simulink model "harvester"  (R2025b)
settings: Solver=FixedStepAuto  StartTime=0.0  StopTime=100  FixedStep=0.1  RelTol=1e-3
values from neighbouring files (symbols this model uses):
  nDrum = 1000    [Script.m]
  nEngine = 2500    [Script.m]
  nHeader = 100    [Script.m]
  sDrum = 1    [Script.m]
  sEngine = 1    [Script.m]
  sGrainConveyor = 1    [Script.m]
  sHeader = 1    [Script.m]
settings Model: Creator=levadny  LastModifiedBy=andr
settings OptimizationCC: DefaultParameterBehavior=Inlined  UseDivisionForNetSlopeComputation=on  OptimizeBlockIOStorage=off  EnhancedBackFolding=on  PassReuseOutputArgsThreshold=0.0  ZeroExternalMemoryAtStartup=off  ZeroInternalMemoryAtStartup=off  OptimizeDataStoreBuffers=off  BusAssignmentInplaceUpdate=off
settings DebuggingCC: ParameterTunabilityLossMsg=error  SFUnexpectedBacktrackingDiag=warning  SFNoUnconditionalDefaultTransitionDiag=warning
settings HardwareCC: ProdLongLongMode=on
settings SFSimCC: SimTargetLang=C++  SimDLTargetLibrary=mkl-dnn
settings RTWCC: GenerateReport=on  BuildConfiguration=Debug  LaunchReport=on  TargetLang=C++  GPUComputeCapability=3.5
settings CodeAppCC: ForceParamTrailComments=on  OperatorAnnotations=on  MATLABSourceComments=on  EnableCustomComments=on
settings GRTTargetCC: MultiInstanceErrorCode=Warning  TargetLangStandard=C++20 (ISO)  UtilityFuncGeneration=Shared location  CombineSignalStateStructs=on  CodeInterfacePackaging=C++ class  SubcomponentCodeInterfacePackaging=C++ class  SupportVariableSizeSignals=on

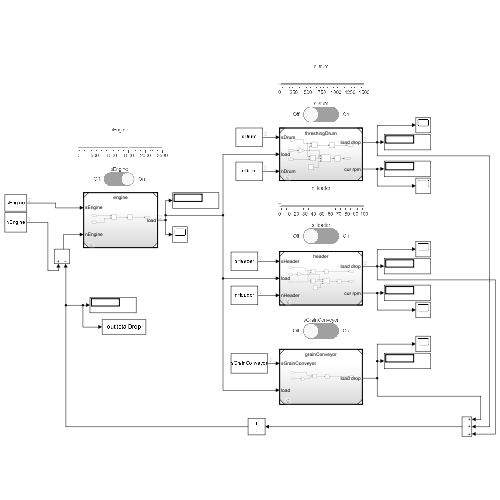
[thumbnail: Simulink's stored preview of the top-level diagram]
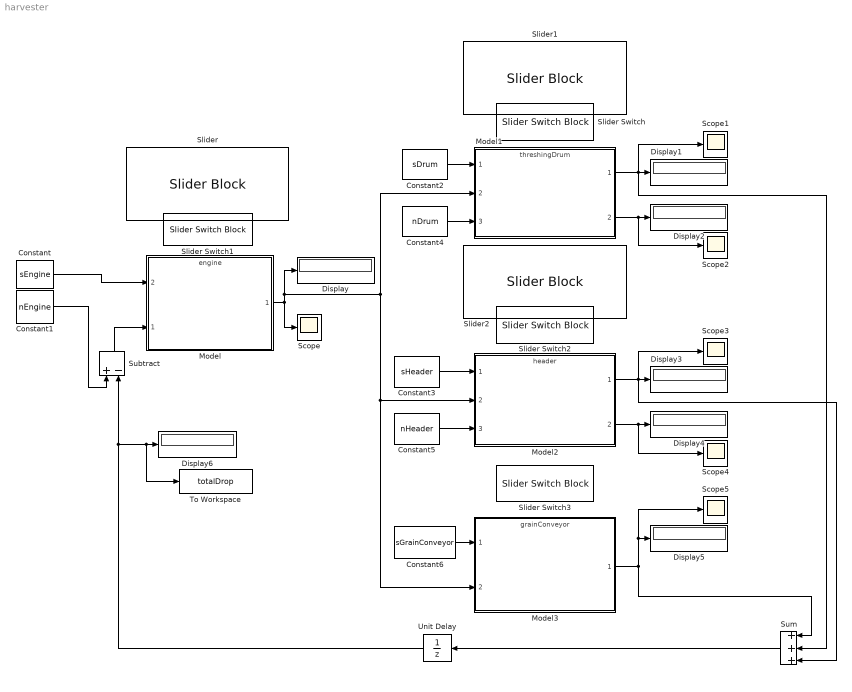
== system harvester ==
  Constant : Constant  Value=sEngine  OutDataTypeStr=boolean
  Constant1 : Constant  Value=nEngine  OutDataTypeStr=double
  Constant2 : Constant  Value=sDrum  OutDataTypeStr=boolean
  Constant3 : Constant  Value=sHeader  OutDataTypeStr=boolean
  Constant4 : Constant  Value=nDrum  OutDataTypeStr=double
  Constant5 : Constant  Value=nHeader  OutDataTypeStr=double
  Constant6 : Constant  Value=sGrainConveyor  OutDataTypeStr=boolean
  Display{,1..6} (7 alike) : Display
  Model : ModelReference  ModelNameDialog=engine.slx  SimulationMode=Normal  ModelReferenceVersion=5.95
      settings: PortSchema="{\"entries\":[{\"content\":{\"sides\":[{\"content\":{\"connectorIds\":[\"In2\",\"In1\"]},\"type\":\"ConnectorPlacement.EquallySpacedRectSide\",\"uuid\":\"37ac5961-e276-4d93-b4c6-6fc5d3558ffa\"},{\"content\":{\"connectorIds\":[\"Out1\"],\"side\":\"RIGHT\"},\"type\":\"ConnectorPlacement.EquallySpacedRectSide\",\"uuid\":\"a95c6b53-13f2-43eb-8466-743c9587078e\"},{\"content\":{\"side\":\"TOP\"},\"type\":\"ConnectorPlacement.EquallySpacedRectSide\",\"uuid\":\"05494b40-a06e-4e30-8915-51b9ee682eaa\"}]},\"type\":\"ConnectorPlacement.EquallySpacedConnector\",\"uuid\":\"41e1e99c-041b-4221-8dab-7a22a8a3a725\"}],\"packageUris\":[\"http://schema.mathworks.com/mf0/Connector/R2020b\"],\"version\":\"1.0\"}"
  Model1 : ModelReference  ModelNameDialog=threshingDrum.slx  SimulationMode=Normal  ModelReferenceVersion=1.110
  Model2 : ModelReference  ModelNameDialog=header.slx  SimulationMode=Normal  ModelReferenceVersion=1.84
  Model3 : ModelReference  ModelNameDialog=grainConveyor.slx  SimulationMode=Normal  ModelReferenceVersion=1.86
  Scope{,1..5} (6 alike) : Scope
      Scope settings: ActiveDisplayYMinimum=-193.74999999999994  ActiveDisplayYMaximum=2243.75
      Scope1 settings: ActiveDisplayYMinimum=-193.74999999999994  ActiveDisplayYMaximum=2243.75
      Scope2 settings: ActiveDisplayYMinimum=-193.74999999999994  ActiveDisplayYMaximum=2243.75  DataLoggingVariableName=ScopeData2
      Scope3 settings: ActiveDisplayYMinimum=-193.74999999999994  ActiveDisplayYMaximum=2243.75  DataLoggingVariableName=ScopeData3
      Scope4 settings: ActiveDisplayYMinimum=-193.74999999999994  ActiveDisplayYMaximum=2243.75  DataLoggingVariableName=ScopeData4
      Scope5 settings: ActiveDisplayYMinimum=-193.74999999999994  ActiveDisplayYMaximum=2243.75  DataLoggingVariableName=ScopeData5
  Slider : SliderBlock  ScaleMax=2500
  Slider Switch{,1..3} (4 alike) : SliderSwitchBlock
  Slider1 : SliderBlock  ScaleMax=1500
  Slider2 : SliderBlock
  Subtract : Sum  Inputs=+-
  Sum : Sum  Inputs=+++
  To Workspace : ToWorkspace  VariableName=totalDrop  SaveFormat=Timeseries  SampleTime=-1
  Unit Delay : UnitDelay  SampleTime=-1  HasFrameUpgradeWarning=on
  wires:
  Constant1/1 -> Subtract/1
  Constant/1 -> Model/2
  Subtract/1 -> Model/1
  Model/1 -> Display/1, Model3/2, Model2/2, Model1/2, Scope/1
  Constant4/1 -> Model1/3
  Constant2/1 -> Model1/1
  Model1/2 -> Scope2/1, Display2/1
  Model1/1 -> Display1/1, Scope1/1, Sum/2
  Unit Delay/1 -> To Workspace/1, Display6/1, Subtract/2
  Model2/2 -> Scope4/1, Display4/1
  Model2/1 -> Sum/3, Scope3/1, Display3/1
  Constant3/1 -> Model2/1
  Constant5/1 -> Model2/3
  Sum/1 -> Unit Delay/1
  Constant6/1 -> Model3/1
  Model3/1 -> Scope5/1, Display5/1, Sum/1
